simulink model "RTdinamicDir"  (R2018a)
settings: Solver=VariableStepAuto  StartTime=0.0  StopTime=10.0  RelTol=1e-3
settings Model: Creator=ilier  LastModifiedBy=ilier

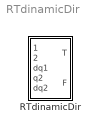
== system RTdinamicDir ==
  RTdinamicDir : Subsystem

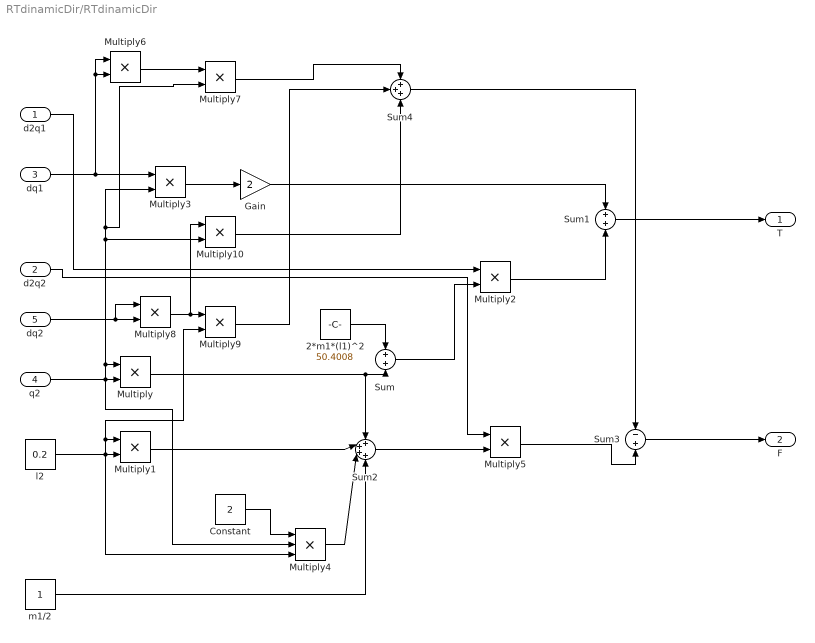
== system RTdinamicDir/RTdinamicDir ==
  d2q1 : Inport
  d2q2 : Inport  Port=2
  dq1 : Inport  Port=3
  q2 : Inport  Port=4
  dq2 : Inport  Port=5
  2*m1*(l1)^2 : Constant  Value=50.4008
  Constant : Constant  Value=2
  Gain : Gain  Gain=2
  Multiply{,1..3,5..10} (10 alike) : Product
  Multiply4 : Product  Inputs=3
  Sum : Sum
  Sum1 : Sum
  Sum2 : Sum  Inputs=++++
  Sum3 : Sum  Inputs=-+
  Sum4 : Sum  Inputs=+++
  l2 : Constant  Value=0.2
  m1/2 : Constant
  T : Outport
  F : Outport  Port=2
  wires:
  Sum3/1 -> F/1
  q2/1 -> Multiply10/2, Multiply7/2, Multiply3/2, Multiply/1, Multiply4/2, Multiply/2
  Multiply2/1 -> Sum1/2
  Multiply1/1 -> Sum2/2
  Sum2/1 -> Multiply5/2
  Sum/1 -> Multiply2/2
  d2q2/1 -> Multiply5/1
  dq1/1 -> Multiply6/2, Multiply6/1, Multiply3/1
  l2/1 -> Multiply1/1, Multiply9/2, Multiply1/2, Multiply4/3
  dq2/1 -> Multiply8/2, Multiply8/1
  Multiply5/1 -> Sum3/2
  Multiply8/1 -> Multiply10/1, Multiply9/1
  Constant/1 -> Multiply4/1
  Multiply3/1 -> Gain/1
  Sum1/1 -> T/1
  2*m1*(l1)^2/1 -> Sum/1
  Multiply7/1 -> Sum4/1
  m1/2/1 -> Sum2/4
  Multiply/1 -> Sum2/1, Sum/2
  Multiply9/1 -> Sum4/2
  Gain/1 -> Sum1/1
  Multiply6/1 -> Multiply7/1
  Multiply10/1 -> Sum4/3
  Sum4/1 -> Sum3/1
  Multiply4/1 -> Sum2/3
  d2q1/1 -> Multiply2/1
